simulink model "Zadatak2PID"  (R2016a)
settings: Solver=VariableStepAuto  SolverMode=SingleTasking  StartTime=0.0  StopTime=300  RelTol=1e-3
values from neighbouring files (symbols this model uses):
  Kp = 1.2*T0/K0/(tau + T) - 0.5*Ki/K0    (= 0.886775962404)    [Parameters.m]
  T = 0.01    [Parameters.m]
  Td = T*Kd/Kp    (= 0.310112149696)    [Parameters.m]
  Ti = Kp*T/Ki    (= 1.46356729475)    [Parameters.m]
libraries: simulink x1
settings Model: Creator=User  LastModifiedBy=M-Pc
settings DebuggingCC: SFUnexpectedBacktrackingDiag=error  SFNoUnconditionalDefaultTransitionDiag=error
settings GRTTargetCC: TargetLangStandard=C99 (ISO)  GeneratePreprocessorConditionals=Use local settings
settings ConfigComp: CovMetricSettings=dwe  CovHtmlReporting=off  CovSaveCumulativeToWorkspaceVar=off  CovSaveSingleToWorkspaceVar=off  CovExternalEMLEnable=on

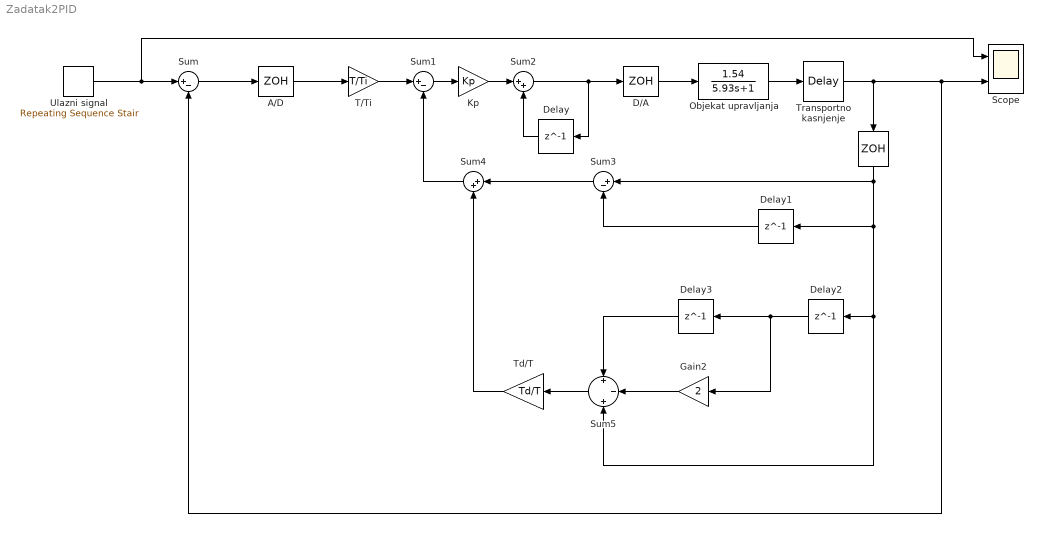
== system Zadatak2PID ==
  " " : ZeroOrderHold  SampleTime=0.01
  A/D : ZeroOrderHold  SampleTime=0.01
  D/A : ZeroOrderHold  SampleTime=0.01
  Delay{,1..3} (4 alike) : Delay  DelayLength=1
  Gain2 : Gain  Gain=2
  Kp : Gain  Gain=Kp
  Objekat upravljanja : TransferFcn  Numerator=[1.54]  Denominator=[5.93 1]
  Scope : Scope  NumInputPorts=2
  Sum : Sum  Inputs=|+-
  Sum1 : Sum  Inputs=|+-
  Sum2 : Sum  Inputs=|++
  Sum3 : Sum  Inputs=|+-
  Sum4 : Sum  Inputs=|++
  Sum5 : Sum  Inputs=+|-|+
  T/Ti : Gain  Gain=T/Ti
  Td/T : Gain  Gain=Td/T
  Transportno kasnjenje : TransportDelay  DelayTime=1.07
  Ulazni signal : simulink/Sources/Repeating Sequence Stair  OutValues=[3 1 -5 2 1].'  tsamp=50  OutMin=[]  OutMax=[]  OutDataTypeStr=double  OutputDataTypeScalingMode=double  OutDataType=fixdt(0,8)  ConRadixGroup=Best Precision: Vector-wise  OutScaling=2^-12
  wires:
  Ulazni signal/1 -> Scope/1, Sum/1
  Sum/1 -> A/D/1
  A/D/1 -> T/Ti/1
  T/Ti/1 -> Sum1/1
  Sum1/1 -> Kp/1
  Kp/1 -> Sum2/1
  Sum2/1 -> Delay/1, D/A/1
  D/A/1 -> Objekat upravljanja/1
  Objekat upravljanja/1 -> Transportno kasnjenje/1
  Delay1/1 -> Sum3/2
  Sum3/1 -> Sum4/1
  Delay2/1 -> Delay3/1, Gain2/1
  Delay3/1 -> Sum5/1
  Gain2/1 -> Sum5/2
  " "/1 -> Sum5/3, Delay2/1, Delay1/1, Sum3/1
  Delay/1 -> Sum2/2
  Sum5/1 -> Td/T/1
  Td/T/1 -> Sum4/2
  Sum4/1 -> Sum1/2
  Transportno kasnjenje/1 -> Sum/2, Scope/2, " "/1
